simulink model "modelo_n_linear0"  (R2013a)
settings: Solver=ode45  StartTime=0.0  StopTime=1  RelTol=1e-3
values from neighbouring files (symbols this model uses):
  dA = [1.435e2 3.335e-2]    [parametriza.m]    (also in parametrizaMancal.m)
  E = 3e9    (= 3000000000)    [parametriza.m]    (also in parametrizaMancal.m)
  Fp_model = fit_Kb    [parametriza.m]
  gb = 0.3e-3    (= 0.0003)    [parametriza.m]    (also in parametrizaMancal.m)
  Hb = 8e-3    (= 0.008)    [parametriza.m]    (also in parametrizaMancal.m)
  Kbb = E*Hb*Ab/Lb    [parametriza.m]
  Kp = 625    [parametriza.m]
  L1 = -1.206e-05    [parametriza.m]
  L2 = 7.807e-05    [parametriza.m]
  Lb = 5.3e-3    (= 0.0053)    [parametriza.m]    (also in parametrizaMancal.m)
  m = 0.375    [parametriza.m]    (also in parametrizaMancal.m)
  R = 6.3    [parametriza.m]    (also in parametrizaMancal.m = 6)
libraries: simulink x2, dspmathops x1
settings Model: Creator=rafa  LastModifiedBy=rafa

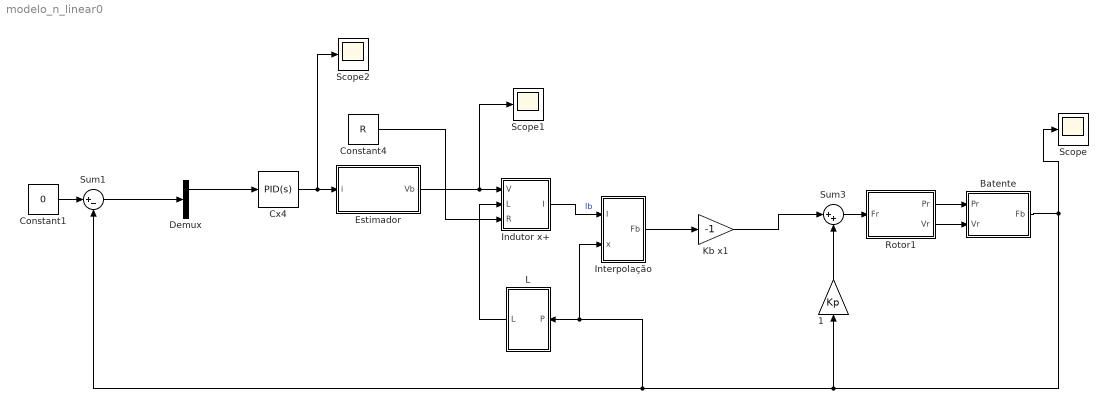
== system modelo_n_linear0 ==
  " 1" : Gain  Gain=Kp
  Batente : Subsystem
  Constant1 : Constant  Value=0
  Constant4 : Constant  Value=R
  Cx4 : simulink/Continuous/PID Controller  Controller=PID  TimeDomain=Continuous-time  SampleTime=1  IntegratorMethod=Forward Euler  FilterMethod=Forward Euler  Form=Ideal  P=631928.6408176  I=23.9651146885149  D=0.00498268867902985  N=6755.34339596169  InitialConditionSource=internal  InitialConditionForIntegrator=0  InitialConditionForFilter=0  ExternalReset=none  LimitOutput=off  UpperSaturationLimit=inf  LowerSaturationLimit=-inf  LinearizeAsGain=on  AntiWindupMode=none  Kb=1  TrackingMode=off  Kt=1  PParamMin=[]  PParamMax=[]  IParamMin=[]  IParamMax=[]  DParamMin=[]  DParamMax=[]  NParamMin=[]  NParamMax=[]  KbParamMin=[]  KbParamMax=[]  KtParamMin=[]  KtParamMax=[]  POutMin=[]  POutMax=[]  IOutMin=[]  IOutMax=[]  DOutMin=[]  DOutMax=[]  NOutMin=[]  NOutMax=[]  KbOutMin=[]  KbOutMax=[]  KtOutMin=[]  KtOutMax=[]  IntegratorOutMin=[]  IntegratorOutMax=[]  FilterOutMin=[]  FilterOutMax=[]  SumOutMin=[]  SumOutMax=[]  SumI1OutMin=[]  SumI1OutMax=[]  SumI2OutMin=[]  SumI2OutMax=[]  SumI3OutMin=[]  SumI3OutMax=[]  SumDOutMin=[]  SumDOutMax=[]  SaturationOutMin=[]  SaturationOutMax=[]  IntegratorContinuousStateAttributes=''  IntegratorStateMustResolveToSignalObject=off  IntegratorRTWStateStorageClass=Auto  FilterContinuousStateAttributes=''  FilterStateMustResolveToSignalObject=off  FilterRTWStateStorageClass=Auto
  Demux : Demux  Outputs=2
  Estimador : Subsystem
  Indutor x+ : Subsystem
  Interpolação : Subsystem
  Kb x1 : Gain  Gain=-1
  L : Subsystem
  Rotor1 : Subsystem
  Scope : Scope
      settings: YMin=-5e-05  YMax=0.0003
  Scope1 : Scope
      settings: YMin=-0.000315  YMax=-0.000285
  Scope2 : Scope
      settings: YMin=-0.000315  YMax=-0.000285  SaveName=ScopeData2
  Sum1 : Sum  Inputs=|+-
  Sum3 : Sum  Inputs=|++
  wires:
  Constant4/1 -> Indutor x+/3(R)
  L/1(L) -> Indutor x+/2(L)
  Kb x1/1 -> Sum3/1
  Sum3/1 -> Rotor1/1(Fr)
  " 1"/1 -> Sum3/2
  Estimador/1(Vb) -> Scope1/1, Indutor x+/1(V)
  Cx4/1 -> Scope2/1, Estimador/1("i ")
  Rotor1/1(Pr) -> Batente/1(Pr)
  Demux/1 -> Cx4/1
  Batente/1(Fb) -> Scope/1, Sum1/2, Interpolação/2(x), L/1(P), " 1"/1
  Indutor x+/1(I) -> Interpolação/1(I)  "Ib"
  Interpolação/1(Fb) -> Kb x1/1
  Sum1/1 -> Demux/1
  Constant1/1 -> Sum1/1
  Rotor1/2(Vr) -> Batente/2(Vr)

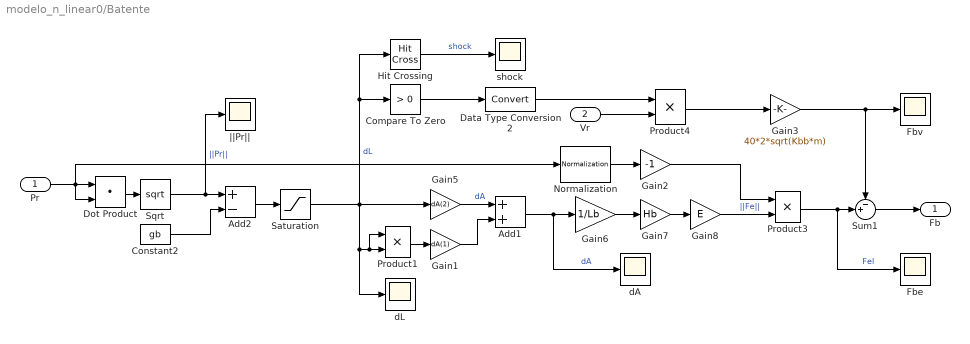
== system modelo_n_linear0/Batente ==
  Pr : Inport
  Vr : Inport  Port=2
  Add1 : Sum
  Add2 : Sum  Inputs=+-
  Compare To Zero : simulink/Logic and Bit Operations/Compare To Zero  relop=>  OutDataTypeStr=boolean
  Constant2 : Constant  Value=gb
  Data Type Conversion2 : DataTypeConversion
  Dot Product : DotProduct  InputSameDT=on  OutDataTypeStr=Inherit: Inherit via internal rule
  Fbe : Scope
      settings: TimeRange=0.0002829354553492485  YMin=-100000  YMax=100000  SaveName=ScopeData15
  Fbv : Scope
      settings: TimeRange=0.1  YMin=-225000  YMax=225000  SaveName=ScopeData8
  Gain1 : Gain  Gain=dA(1)
  Gain2 : Gain  Gain=-1
  Gain3 : Gain  Gain=40*2*sqrt(Kbb*m)
  Gain5 : Gain  Gain=dA(2)
  Gain6 : Gain  Gain=1/Lb
  Gain7 : Gain  Gain=Hb
  Gain8 : Gain  Gain=E
  Hit Crossing : HitCross  HitCrossingDirection=rising
  Normalization : dspmathops/Normalization  NormType=2-norm  Bias=1e-10  NormOver=Each column  ColComp=on  Dimension=1  outputDataTypeStr=Inherit: Same as product output  outputLastDataTypeStr=Inherit: Same as product output  outputMin=[]  outputMax=[]  accumDataTypeStr=Inherit: Same as product output  accumLastDataTypeStr=Inherit: Same as product output  roundingMode=Floor  overflowMode=off
  Product1 : Product
  Product3 : Product
  Product4 : Product
  Saturation : Saturate  UpperLimit=Inf  LowerLimit=0
  Sqrt : Sqrt  SaturateOnIntegerOverflow=on
  Sum1 : Sum  Inputs=-+|
  dA : Scope
      settings: TimeRange=0.0002829354553492485  YMin=3.91545e-05  YMax=3.9158e-05  SaveName=ScopeData4
  dL : Scope
      settings: TimeRange=0.1  YMin=1.4215e-06  YMax=1.4315e-06  SaveName=ScopeData7
  shock : Scope
      settings: TimeRange=0.0002829354553492485  YMin=5.54637e-16  YMax=5.54639e-16  SaveName=ScopeData19
  ||Pr|| : Scope
      settings: TimeRange=0.0002829354553492485  YMin=-2.75  YMax=0  SaveName=ScopeData18
  Fb : Outport
  wires:
  Dot Product/1 -> Sqrt/1
  Gain8/1 -> Product3/2  "||Fe||"
  Compare To Zero/1 -> Data Type Conversion2/1
  Saturation/1 -> dL/1, Product1/1, Product1/2, Hit Crossing/1, Compare To Zero/1, Gain5/1  "dL"
  Add2/1 -> Saturation/1
  Sqrt/1 -> ||Pr||/1, Add2/1  "||Pr||"
  Constant2/1 -> Add2/2
  Gain6/1 -> Gain7/1
  Gain7/1 -> Gain8/1
  Product4/1 -> Gain3/1
  Product3/1 -> Sum1/2, Fbe/1  "Fel"
  Sum1/1 -> Fb/1
  Data Type Conversion2/1 -> Product4/1
  Product1/1 -> Gain1/1
  Gain5/1 -> Add1/1  "dA"
  Add1/1 -> dA/1, Gain6/1  "dA"
  Gain3/1 -> Fbv/1, Sum1/1
  Vr/1 -> Product4/2
  Normalization/1 -> Gain2/1
  Pr/1 -> Normalization/1, Dot Product/2, Dot Product/1
  Gain2/1 -> Product3/1
  Gain1/1 -> Add1/2
  Hit Crossing/1 -> shock/1  "shock"

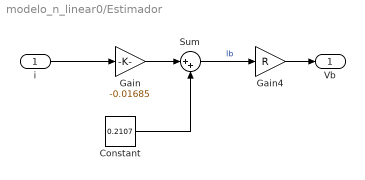
== system modelo_n_linear0/Estimador ==
  "i " : Inport
  Constant : Constant  Value=0.2107
  Gain : Gain  Gain=-0.01685
  Gain4 : Gain  Gain=R
  Sum : Sum  Inputs=|++
  Vb : Outport
  wires:
  Gain4/1 -> Vb/1
  Sum/1 -> Gain4/1  "Ib"
  "i "/1 -> Gain/1
  Gain/1 -> Sum/1
  Constant/1 -> Sum/2

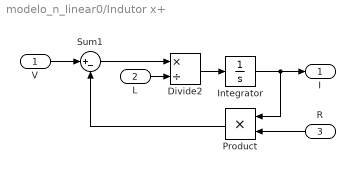
== system modelo_n_linear0/Indutor x+ ==
  V : Inport
  L : Inport  Port=2
  R : Inport  Port=3
  Divide2 : Product  Inputs=*/
  Integrator : Integrator
  Product : Product
  Sum1 : Sum  Inputs=|+-
  I : Outport
  wires:
  Divide2/1 -> Integrator/1
  Sum1/1 -> Divide2/1
  Integrator/1 -> Product/1, I/1
  Product/1 -> Sum1/2
  L/1 -> Divide2/2
  V/1 -> Sum1/1
  R/1 -> Product/2

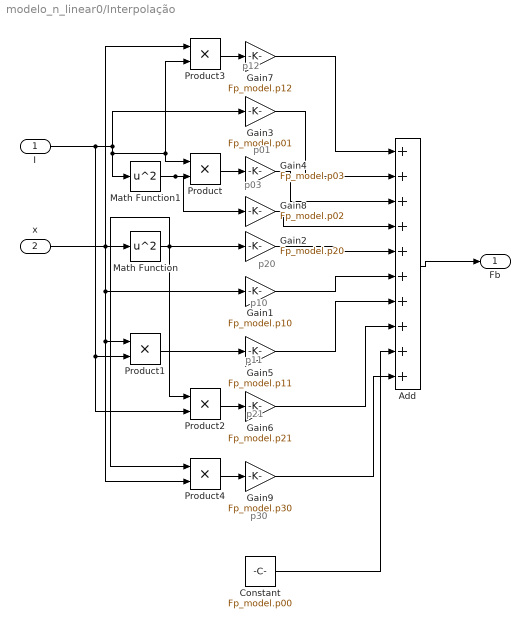
== system modelo_n_linear0/Interpolação ==
  note: p12
  note: p01
  note: p20
  note: p10
  note: p11
  note: p21
  note: p30
  note: p03
  I : Inport
  x : Inport  Port=2
  Add : Sum  Inputs=++++++++++
  Constant : Constant  Value=Fp_model.p00
  Gain1 : Gain  Gain=Fp_model.p10
  Gain2 : Gain  Gain=Fp_model.p20
  Gain3 : Gain  Gain=Fp_model.p01
  Gain4 : Gain  Gain=Fp_model.p03
  Gain5 : Gain  Gain=Fp_model.p11
  Gain6 : Gain  Gain=Fp_model.p21
  Gain7 : Gain  Gain=Fp_model.p12
  Gain8 : Gain  Gain=Fp_model.p02
  Gain9 : Gain  Gain=Fp_model.p30
  Math Function : Math  Operator=square  SaturateOnIntegerOverflow=on
  Math Function1 : Math  Operator=square  SaturateOnIntegerOverflow=on
  Product{,1..4} (5 alike) : Product  RndMeth=Zero
  Fb : Outport
  wires:
  I/1 -> Product2/2, Product1/2, Gain3/1, Math Function1/1, Product/1, Product3/2
  Product/1 -> Gain4/1
  Math Function1/1 -> Gain8/1, Product/2
  Gain4/1 -> Add/3
  x/1 -> Product3/1, Product4/2, Product1/1, Gain1/1, Math Function/1
  Math Function/1 -> Product4/1, Product2/1, Gain2/1
  Product1/1 -> Gain5/1
  Product2/1 -> Gain6/1
  Product3/1 -> Gain7/1
  Constant/1 -> Add/9
  Gain7/1 -> Add/1
  Gain3/1 -> Add/2
  Gain8/1 -> Add/4
  Gain2/1 -> Add/5
  Gain1/1 -> Add/6
  Gain5/1 -> Add/7
  Gain6/1 -> Add/8
  Add/1 -> Fb/1
  Product4/1 -> Gain9/1
  Gain9/1 -> Add/10

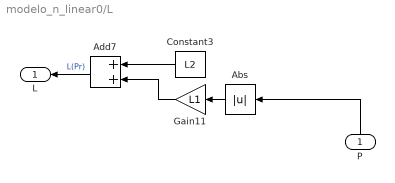
== system modelo_n_linear0/L ==
  P : Inport
  Abs : Abs
  Add7 : Sum
  Constant3 : Constant  Value=L2
  Gain11 : Gain  Gain=L1
  L : Outport
  wires:
  P/1 -> Abs/1
  Add7/1 -> L/1  "L(Pr)"
  Constant3/1 -> Add7/1
  Gain11/1 -> Add7/2
  Abs/1 -> Gain11/1

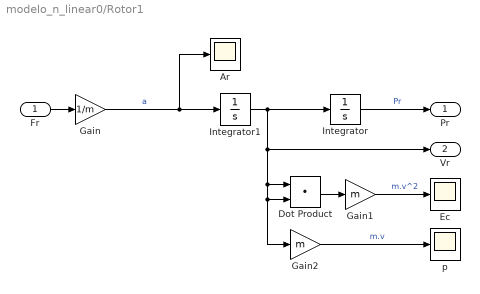
== system modelo_n_linear0/Rotor1 ==
  Fr : Inport
  Ar : Scope
      settings: TimeRange=1  YMin=-200000  YMax=200000  SaveName=ScopeData9
  Dot Product : DotProduct  InputSameDT=on  OutDataTypeStr=Inherit: Inherit via internal rule
  Ec : Scope
      settings: TimeRange=0.25  YMin=0  YMax=0.09  SaveName=ScopeData16
  Gain : Gain  Gain=1/m
  Gain1 : Gain  Gain=m
  Gain2 : Gain  Gain=m
  Integrator : Integrator  InitialCondition=[.001 .002]*1e-3  UpperSaturationLimit=Inf  LowerSaturationLimit=-Inf
  Integrator1 : Integrator
  p : Scope
      settings: TimeRange=1  YMin=-200000  YMax=200000  SaveName=ScopeData17
  Pr : Outport
  Vr : Outport  Port=2
  wires:
  Fr/1 -> Gain/1
  Integrator/1 -> Pr/1  "Pr"
  Gain/1 -> Ar/1, Integrator1/1  "a"
  Dot Product/1 -> Gain1/1
  Gain2/1 -> p/1  "m.v"
  Gain1/1 -> Ec/1  "m.v^2"
  Integrator1/1 -> Vr/1, Dot Product/1, Gain2/1, Dot Product/2, Integrator/1
